simulink model "dampening_model"  (R2014a)
settings: Solver=ode3  StartTime=0.0  StopTime=20  FixedStep=.01  RelTol=1e-3
libraries: simulink x1
settings Model: Creator=wheelerj  LastModifiedBy=wheelerj

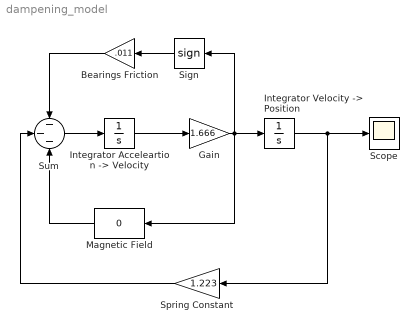
== system dampening_model ==
  Bearings Friction : Gain  Gain=.011
  Gain : Gain  Gain=1.666
  "Integrator Acceleartion -> Velocity" : Integrator
  "Integrator Velocity -> Position " : Integrator  InitialCondition=-.4
  Magnetic Field : simulink/Math Operations/Slider Gain  low=0  gain=0  high=3
  Scope : Scope
      settings: TimeRange=20  YMin=-0.4  YMax=0.1  Decimation=10
  Sign : Signum
  "Spring Constant " : Gain  Gain=1.223
  Sum : Sum  Inputs=---
  wires:
  "Integrator Velocity -> Position "/1 -> "Spring Constant "/1, Scope/1
  Sum/1 -> "Integrator Acceleartion -> Velocity"/1
  Sign/1 -> Bearings Friction/1
  Magnetic Field/1 -> Sum/3
  Bearings Friction/1 -> Sum/1
  "Integrator Acceleartion -> Velocity"/1 -> Gain/1
  Gain/1 -> Sign/1, "Integrator Velocity -> Position "/1, Magnetic Field/1
  "Spring Constant "/1 -> Sum/2
